simulink model "gUSBampDuo"  (R2021a)
settings: Solver=FixedStepDiscrete  StartTime=0.0  StopTime=inf  FixedStep=1/1200  RelTol=1e-3  EnableMultiTasking=on
undefined symbols (not defined in the file or in its folder): currentCFG_gUSBampDuo_UB, UB
libraries: gUSBamplib x2, Tools x1, gtecHighspeedLib x1
settings Model: Creator=gtec  LastModifiedBy=kotani
settings SolverCC: AlgebraicLoopSolver=TrustRegion
settings DataIOCC: LimitDataPoints=on  SaveFormat=Array  ReturnWorkspaceOutputs=off
settings OptimizationCC: LifeSpan=inf
settings DebuggingCC: SolverPrmCheckMsg=warning  SFUnexpectedBacktrackingDiag=warning  SFNoUnconditionalDefaultTransitionDiag=warning  SFExecutionAtInitializationDiag=none  SFMachineParentedDataDiag=warning  ArithmeticOperatorsInVariantConditions=warning
settings HardwareCC: ProdBitPerPointer=32  ProdBitPerSizeT=32  ProdBitPerPtrDiffT=32  ProdLargestAtomicFloat=None  ProdIntDivRoundTo=Undefined  ProdEndianess=Unspecified  ProdWordSize=32  ProdHWDeviceType=32-bit Generic
settings ModelReferenceCC: PropagateSignalLabelsOutOfModel=off
settings SFSimCC: SimUseLocalCustomCode=off  CustomCodeUndefinedFunction=UseInterfaceOnly
settings RTWCC: RTWUseLocalCustomCode=off
settings CodeAppCC: StateflowObjectComments=on
settings GRTTargetCC: TargetLangStandard=C89/C90 (ANSI)
settings ConfigComp: CovMetricSettings=dw  CovSaveCumulativeToWorkspaceVar=on  CovSaveSingleToWorkspaceVar=on  CovExternalEMLEnable=off  CovSFcnEnable=off

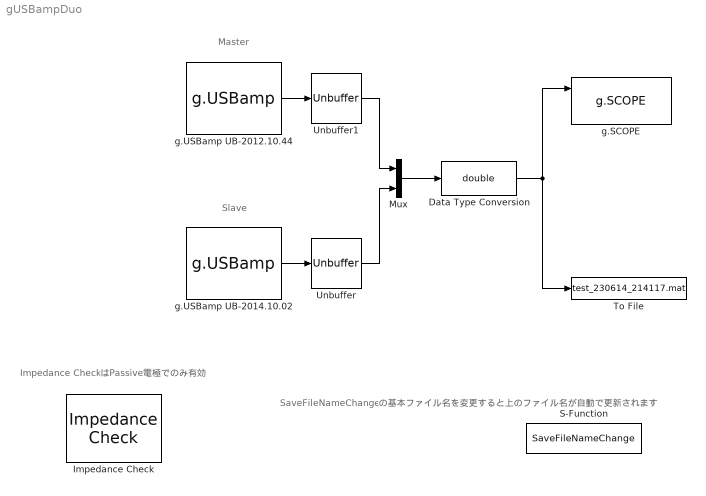
== system gUSBampDuo ==
  note: Impedance CheckはPassive電極でのみ有効
  note: Slave
  note: Master
  note: SaveFileNameChangeの基本ファイル名を変更すると上のファイル名が自動で更新されます
  Data Type Conversion : DataTypeConversion  OutDataTypeStr=double
  Impedance Check : Tools/Impedance Check
  Mux : Mux  Inputs=2
  S-Function : S-Function  FunctionName=SaveFileNameChange  Parameters=modelname,savename  SFunctionDeploymentMode=off  EnableBusSupport=off  mask{modelname=To File, savename=test}
      mask prompts: modelname "To Fileのモデル名"; savename "基本ファイル名"
  To File : ToFile  Filename=test_230614_214117.mat  MatrixName=y
  Unbuffer : Unbuffer
  Unbuffer1 : Unbuffer
  g.SCOPE : gtecHighspeedLib/g.SCOPE
      settings: SourceProductName=g.tec Highspeed Library
  g.USBamp UB-2012.10.44 : gUSBamplib/g.USBamp  Priority=2  cfg=currentCFG_gUSBampDuo_UB-2012.10.44.cfg  snr=UB-2012.10.44
      settings: SourceProductName=g.USBamp
  g.USBamp UB-2014.10.02 : gUSBamplib/g.USBamp  Priority=1  cfg=currentCFG_gUSBampDuo_UB-2014.10.02.cfg  snr=UB-2014.10.02
      settings: SourceProductName=g.USBamp
  wires:
  Data Type Conversion/1 -> To File/1, g.SCOPE/1
  g.USBamp UB-2014.10.02/1 -> Unbuffer/1
  g.USBamp UB-2012.10.44/1 -> Unbuffer1/1
  Unbuffer1/1 -> Mux/1
  Unbuffer/1 -> Mux/2
  Mux/1 -> Data Type Conversion/1
